simulink model "adjust_error_shaped"  (Simulink 8.1)
settings: Solver=ode45  StartTime=0.0  StopTime=10.0  RelTol=1e-3
libraries: simulink x1
settings Model: Creator=Kostas  LastModifiedBy=Kostas
settings DataIOCC: SignalLoggingSaveFormat=Dataset
settings OptimizationCC: ExpressionDepthLimit=128
settings DebuggingCC: FcnCallInpInsideContextMsg=EnableAllAsError
settings GRTTargetCC: CombineOutputUpdateFcns=on  GRTInterface=off

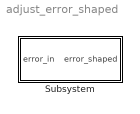
== system adjust_error_shaped ==
  Subsystem : Subsystem

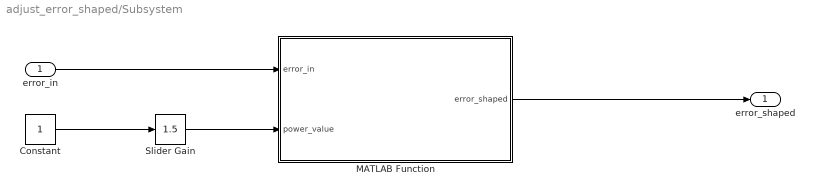
== system adjust_error_shaped/Subsystem ==
  error_in : Inport
  Constant : Constant
  MATLAB Function : MATLAB Function  TreatAsAtomicUnit=on
  Slider Gain : simulink/Math Operations/Slider Gain  low=0  gain=1.5  high=2
  error_shaped : Outport
  wires:
  error_in/1 -> MATLAB Function/1(error_in)
  MATLAB Function/1(error_shaped) -> error_shaped/1
  Slider Gain/1 -> MATLAB Function/2(power_value)
  Constant/1 -> Slider Gain/1

== matlab function Subsystem/MATLAB Function ==
  data: error_in input double; error_shaped output double; power_value input double
function error_shaped = error_shaper(error_in,power_value)
%#codegen

error_shaped = abs(error_in)^power_value;
if error_in < 0
    error_shaped = - error_in;
end

end
